simulink model "uz_interlockDeadtime2L"  (R2023a)
settings: Solver=FixedStepDiscrete  StartTime=0.0  StopTime=0.003  RelTol=1e-3
undefined symbols (not defined in the file or in its folder): f_FPGA_clk, T_FPGA_clk
libraries: simulink x3, hdlsllib x3
(part 2 of 2)

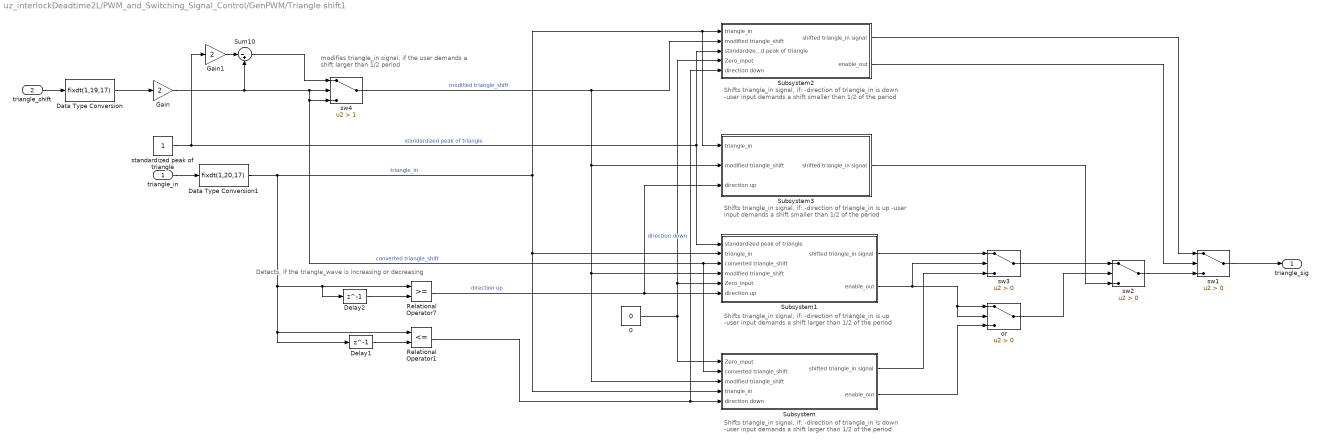
== system uz_interlockDeadtime2L/PWM_and_Switching_Signal_Control/GenPWM/Triangle shift1 ==
  note: modifies triangle_in signal,
      | if the user demands a shift larger than 1/2 period
  note: Detects, if the triangle_wave is increasing or decreasing
  note: Shifts triangle_in signal, if:
      | -direction of triangle_in is down
      | -user input demands a shift larger than 1/2 of the period
  note: Shifts triangle_in signal, if:
      | -direction of triangle_in is up
      | -user input demands a shift larger than 1/2 of the period
  note: Shifts triangle_in signal, if:
      | -direction of triangle_in is up
      | -user input demands a shift smaller than 1/2 of the period
  note: Shifts triangle_in signal, if:
      | -direction of triangle_in is down
      | -user input demands a shift smaller than 1/2 of the period
  triangle_in : Inport
  triangle_shift : Inport  Port=2
  0 : Constant  Value=0  OutDataTypeStr=boolean  SampleTime=T_FPGA_clk
  Data Type Conversion : DataTypeConversion  OutDataTypeStr=fixdt(1,19,17)  SaturateOnIntegerOverflow=off  RndMeth=Floor
  Data Type Conversion1 : DataTypeConversion  OutDataTypeStr=fixdt(1,20,17)  SaturateOnIntegerOverflow=off  RndMeth=Floor
  Delay1 : Delay  DelayLength=1
  Delay2 : Delay  DelayLength=1
  Gain : Gain  Gain=2  OutDataTypeStr=fixdt(1,20,17)
  Gain1 : Gain  Gain=2  OutDataTypeStr=fixdt(1,20,17)
  Relational Operator1 : RelationalOperator  Operator=<=  OutDataTypeStr=boolean  InputSameDT=off
  Relational Operator7 : RelationalOperator  OutDataTypeStr=boolean  InputSameDT=off
  Subsystem : Subsystem
  Subsystem1 : Subsystem
  Subsystem2 : Subsystem
  Subsystem3 : Subsystem
  Sum10 : Sum  Inputs=|-+  OutDataTypeStr=fixdt(1,20,17)
  or : Switch  Criteria=u2 > Threshold  SaturateOnIntegerOverflow=off  InputSameDT=off
  standardized peak of triangle : Constant  OutDataTypeStr=fixdt(0,21,17)  SampleTime=T_FPGA_clk
  sw1 : Switch  Criteria=u2 > Threshold  OutDataTypeStr=fixdt(1,18,16)  SaturateOnIntegerOverflow=off  InputSameDT=off
  sw2 : Switch  Criteria=u2 > Threshold  SaturateOnIntegerOverflow=off  InputSameDT=off
  sw3 : Switch  Criteria=u2 > Threshold  SaturateOnIntegerOverflow=off  InputSameDT=off
  sw4 : Switch  Criteria=u2 > Threshold  Threshold=1  OutDataTypeStr=fixdt(1,20,17)  SaturateOnIntegerOverflow=off  InputSameDT=off
  triangle_sig : Outport  VectorParamsAs1DForOutWhenUnconnected=off
  wires:
  Delay2/1 -> Relational Operator7/2
  Data Type Conversion1/1 -> Subsystem3/1(triangle_in), Subsystem2/1(triangle_in), Subsystem/4(triangle_in), Subsystem1/2(triangle_in), Relational Operator1/1, Delay1/1, Delay2/1, Relational Operator7/1  "triangle_in"
  sw3/1 -> sw2/1
  Relational Operator7/1 -> Subsystem1/6(direction up), Subsystem3/3(direction up)  "direction up"
  or/1 -> sw2/2
  sw4/1 -> Subsystem3/2(modified triangle_shift), Subsystem/3(modified triangle_shift), Subsystem1/4(modified triangle_shift), Subsystem2/2(modified triangle_shift)  "modified triangle_shift"
  Gain/1 -> Sum10/2, Subsystem/2(converted triangle_shift), Subsystem1/3(converted triangle_shift), sw4/3, sw4/2  "converted triangle_shift"
  Sum10/1 -> sw4/1
  sw1/1 -> triangle_sig/1
  standardized peak of triangle/1 -> Subsystem2/3(standardized peak of triangle), Subsystem1/1(standardized peak of triangle), Gain1/1  "standardized peak of triangle"
  triangle_shift/1 -> Data Type Conversion/1
  Gain1/1 -> Sum10/1
  sw2/1 -> sw1/3
  Data Type Conversion/1 -> Gain/1
  triangle_in/1 -> Data Type Conversion1/1
  Relational Operator1/1 -> Subsystem/5(direction down), Subsystem2/5(direction down)  "direction down"
  Delay1/1 -> Relational Operator1/2
  0/1 -> Subsystem2/4(Zero_input), Subsystem1/5(Zero_input), Subsystem/1(Zero_input)
  Subsystem/1(shifted triangle_in signal) -> sw3/3
  Subsystem/2(enable_out) -> or/3
  Subsystem1/2(enable_out) -> or/2, or/1, sw3/2
  Subsystem1/1(shifted triangle_in signal) -> sw3/1
  Subsystem2/1(shifted triangle_in signal) -> sw1/1
  Subsystem2/2(enable_out) -> sw1/2
  Subsystem3/1(shifted triangle_in signal) -> sw2/3

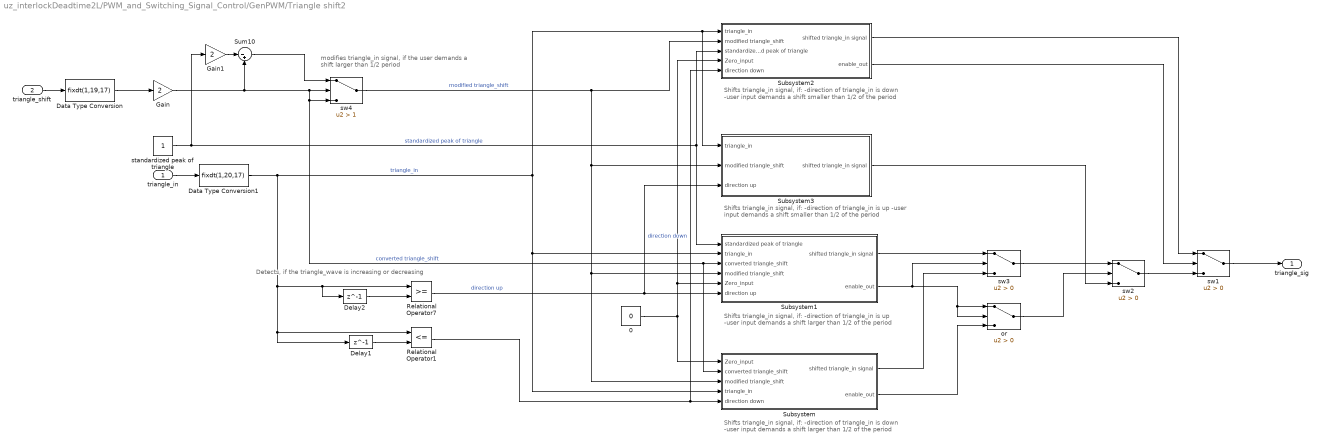
== system uz_interlockDeadtime2L/PWM_and_Switching_Signal_Control/GenPWM/Triangle shift2 ==
  note: modifies triangle_in signal,
      | if the user demands a shift larger than 1/2 period
  note: Detects, if the triangle_wave is increasing or decreasing
  note: Shifts triangle_in signal, if:
      | -direction of triangle_in is down
      | -user input demands a shift larger than 1/2 of the period
  note: Shifts triangle_in signal, if:
      | -direction of triangle_in is up
      | -user input demands a shift larger than 1/2 of the period
  note: Shifts triangle_in signal, if:
      | -direction of triangle_in is up
      | -user input demands a shift smaller than 1/2 of the period
  note: Shifts triangle_in signal, if:
      | -direction of triangle_in is down
      | -user input demands a shift smaller than 1/2 of the period
  triangle_in : Inport
  triangle_shift : Inport  Port=2
  0 : Constant  Value=0  OutDataTypeStr=boolean  SampleTime=T_FPGA_clk
  Data Type Conversion : DataTypeConversion  OutDataTypeStr=fixdt(1,19,17)  SaturateOnIntegerOverflow=off  RndMeth=Floor
  Data Type Conversion1 : DataTypeConversion  OutDataTypeStr=fixdt(1,20,17)  SaturateOnIntegerOverflow=off  RndMeth=Floor
  Delay1 : Delay  DelayLength=1
  Delay2 : Delay  DelayLength=1
  Gain : Gain  Gain=2  OutDataTypeStr=fixdt(1,20,17)
  Gain1 : Gain  Gain=2  OutDataTypeStr=fixdt(1,20,17)
  Relational Operator1 : RelationalOperator  Operator=<=  OutDataTypeStr=boolean  InputSameDT=off
  Relational Operator7 : RelationalOperator  OutDataTypeStr=boolean  InputSameDT=off
  Subsystem : Subsystem
  Subsystem1 : Subsystem
  Subsystem2 : Subsystem
  Subsystem3 : Subsystem
  Sum10 : Sum  Inputs=|-+  OutDataTypeStr=fixdt(1,20,17)
  or : Switch  Criteria=u2 > Threshold  SaturateOnIntegerOverflow=off  InputSameDT=off
  standardized peak of triangle : Constant  OutDataTypeStr=fixdt(0,21,17)  SampleTime=T_FPGA_clk
  sw1 : Switch  Criteria=u2 > Threshold  OutDataTypeStr=fixdt(1,18,16)  SaturateOnIntegerOverflow=off  InputSameDT=off
  sw2 : Switch  Criteria=u2 > Threshold  SaturateOnIntegerOverflow=off  InputSameDT=off
  sw3 : Switch  Criteria=u2 > Threshold  SaturateOnIntegerOverflow=off  InputSameDT=off
  sw4 : Switch  Criteria=u2 > Threshold  Threshold=1  OutDataTypeStr=fixdt(1,20,17)  SaturateOnIntegerOverflow=off  InputSameDT=off
  triangle_sig : Outport  VectorParamsAs1DForOutWhenUnconnected=off
  wires:
  Delay2/1 -> Relational Operator7/2
  Data Type Conversion1/1 -> Subsystem3/1(triangle_in), Subsystem2/1(triangle_in), Subsystem/4(triangle_in), Subsystem1/2(triangle_in), Relational Operator1/1, Delay1/1, Delay2/1, Relational Operator7/1  "triangle_in"
  sw3/1 -> sw2/1
  Relational Operator7/1 -> Subsystem1/6(direction up), Subsystem3/3(direction up)  "direction up"
  or/1 -> sw2/2
  sw4/1 -> Subsystem3/2(modified triangle_shift), Subsystem/3(modified triangle_shift), Subsystem1/4(modified triangle_shift), Subsystem2/2(modified triangle_shift)  "modified triangle_shift"
  Gain/1 -> Sum10/2, Subsystem/2(converted triangle_shift), Subsystem1/3(converted triangle_shift), sw4/3, sw4/2  "converted triangle_shift"
  Sum10/1 -> sw4/1
  sw1/1 -> triangle_sig/1
  standardized peak of triangle/1 -> Subsystem2/3(standardized peak of triangle), Subsystem1/1(standardized peak of triangle), Gain1/1  "standardized peak of triangle"
  triangle_shift/1 -> Data Type Conversion/1
  Gain1/1 -> Sum10/1
  sw2/1 -> sw1/3
  Data Type Conversion/1 -> Gain/1
  triangle_in/1 -> Data Type Conversion1/1
  Relational Operator1/1 -> Subsystem/5(direction down), Subsystem2/5(direction down)  "direction down"
  Delay1/1 -> Relational Operator1/2
  0/1 -> Subsystem2/4(Zero_input), Subsystem1/5(Zero_input), Subsystem/1(Zero_input)
  Subsystem/1(shifted triangle_in signal) -> sw3/3
  Subsystem/2(enable_out) -> or/3
  Subsystem1/2(enable_out) -> or/2, or/1, sw3/2
  Subsystem1/1(shifted triangle_in signal) -> sw3/1
  Subsystem2/1(shifted triangle_in signal) -> sw1/1
  Subsystem2/2(enable_out) -> sw1/2
  Subsystem3/1(shifted triangle_in signal) -> sw2/3

== system uz_interlockDeadtime2L/PWM_and_Switching_Signal_Control/GenPWM/Triangle shift/Subsystem ==
  note: AND block replaced with
      | switches for better performance
  Zero_input : Inport
  converted triangle_shift : Inport  Port=2
  modified triangle_shift : Inport  Port=3
  triangle_in : Inport  Port=4
  direction down : Inport  Port=5
  Relational Operator11 : RelationalOperator  Operator=<=  OutDataTypeStr=boolean  InputSameDT=off
  Sum8 : Sum  Inputs=|-+
  Unary Minus : UnaryMinus
  and2_1 : Switch  Criteria=u2 > Threshold  SaturateOnIntegerOverflow=off  InputSameDT=off
  and2_2 : Switch  Criteria=u2 > Threshold  SaturateOnIntegerOverflow=off  InputSameDT=off
  shifted triangle_in signal : Outport
  enable_out : Outport  Port=2
  wires:
  direction down/1 -> and2_2/2
  Zero_input/1 -> and2_1/3, and2_2/3
  Relational Operator11/1 -> and2_1/2
  and2_1/1 -> and2_2/1
  Sum8/1 -> shifted triangle_in signal/1
  Unary Minus/1 -> Sum8/2, Relational Operator11/2
  triangle_in/1 -> Sum8/1, Relational Operator11/1
  converted triangle_shift/1 -> and2_1/1
  and2_2/1 -> enable_out/1
  modified triangle_shift/1 -> Unary Minus/1

== system uz_interlockDeadtime2L/PWM_and_Switching_Signal_Control/GenPWM/Triangle shift/Subsystem1 ==
  note: AND block replaced with
      | switches for better performance
  note: AND block replaced with
      | switches for better performance
  standardized peak of triangle : Inport
  triangle_in : Inport  Port=2
  converted triangle_shift : Inport  Port=3
  modified triangle_shift : Inport  Port=4
  Zero_input : Inport  Port=5
  direction up : Inport  Port=6
  Relational Operator2 : RelationalOperator  OutDataTypeStr=boolean  InputSameDT=off
  Sum11 : Sum  Inputs=++-  OutDataTypeStr=fixdt(1,21,17)
  Sum6 : Sum  Inputs=++|
  and1_1 : Switch  Criteria=u2 > Threshold  SaturateOnIntegerOverflow=off  InputSameDT=off
  and1_2 : Switch  Criteria=u2 > Threshold  SaturateOnIntegerOverflow=off  InputSameDT=off
  shifted triangle_in signal : Outport
  enable_out : Outport  Port=2
  wires:
  Sum11/1 -> shifted triangle_in signal/1
  Sum6/1 -> Relational Operator2/2, Sum11/2
  and1_1/1 -> and1_2/1
  Relational Operator2/1 -> and1_1/2
  Zero_input/1 -> and1_2/3, and1_1/3
  standardized peak of triangle/1 -> Sum6/2, Sum11/1
  and1_2/1 -> enable_out/1
  converted triangle_shift/1 -> and1_1/1
  direction up/1 -> and1_2/2
  triangle_in/1 -> Relational Operator2/1, Sum11/3
  modified triangle_shift/1 -> Sum6/1

== system uz_interlockDeadtime2L/PWM_and_Switching_Signal_Control/GenPWM/Triangle shift/Subsystem2 ==
  triangle_in : Inport
  modified triangle_shift : Inport  Port=2
  standardized peak of triangle : Inport  Port=3
  Zero_input : Inport  Port=4
  direction down : Inport  Port=5
  Relational Operator9 : RelationalOperator  OutDataTypeStr=boolean  InputSameDT=off
  Sum1 : Sum  Inputs=|-+
  Sum5 : Sum  Inputs=++-  OutDataTypeStr=fixdt(1,21,17)
  and : Switch  Criteria=u2 > Threshold  SaturateOnIntegerOverflow=off  InputSameDT=off
  shifted triangle_in signal : Outport
  enable_out : Outport  Port=2
  wires:
  standardized peak of triangle/1 -> Sum1/2, Sum5/2
  Zero_input/1 -> and/3
  Sum1/1 -> Relational Operator9/2, Sum5/1
  Relational Operator9/1 -> and/1
  direction down/1 -> and/2
  and/1 -> enable_out/1
  triangle_in/1 -> Relational Operator9/1, Sum5/3
  Sum5/1 -> shifted triangle_in signal/1
  modified triangle_shift/1 -> Sum1/1

== system uz_interlockDeadtime2L/PWM_and_Switching_Signal_Control/GenPWM/Triangle shift/Subsystem3 ==
  triangle_in : Inport
  modified triangle_shift : Inport  Port=2
  direction up : Inport  Port=3
  Relational Operator6 : RelationalOperator  Operator=<=  OutDataTypeStr=boolean  InputSameDT=off
  Sum2 : Sum  Inputs=|-+
  Sum3 : Sum  Inputs=|+-
  Sum4 : Sum  Inputs=|++
  Switch3 : Switch  Criteria=u2 > Threshold  SaturateOnIntegerOverflow=off  InputSameDT=off
  sw : Switch  Criteria=u2 > Threshold  SaturateOnIntegerOverflow=off  InputSameDT=off
  shifted triangle_in signal : Outport
  wires:
  Sum4/1 -> sw/3
  modified triangle_shift/1 -> Sum4/1, Sum3/2, Sum2/2, Relational Operator6/2
  Switch3/1 -> sw/1
  Sum3/1 -> Switch3/3
  Sum2/1 -> Switch3/1
  sw/1 -> shifted triangle_in signal/1
  Relational Operator6/1 -> Switch3/2
  direction up/1 -> sw/2
  triangle_in/1 -> Relational Operator6/1, Sum3/1, Sum2/1, Sum4/2

== system uz_interlockDeadtime2L/PWM_and_Switching_Signal_Control/GenPWM/Triangle shift1/Subsystem ==
  note: AND block replaced with
      | switches for better performance
  Zero_input : Inport
  converted triangle_shift : Inport  Port=2
  modified triangle_shift : Inport  Port=3
  triangle_in : Inport  Port=4
  direction down : Inport  Port=5
  Relational Operator11 : RelationalOperator  Operator=<=  OutDataTypeStr=boolean  InputSameDT=off
  Sum8 : Sum  Inputs=|-+
  Unary Minus : UnaryMinus
  and2_1 : Switch  Criteria=u2 > Threshold  SaturateOnIntegerOverflow=off  InputSameDT=off
  and2_2 : Switch  Criteria=u2 > Threshold  SaturateOnIntegerOverflow=off  InputSameDT=off
  shifted triangle_in signal : Outport
  enable_out : Outport  Port=2
  wires:
  direction down/1 -> and2_2/2
  Zero_input/1 -> and2_1/3, and2_2/3
  Relational Operator11/1 -> and2_1/2
  and2_1/1 -> and2_2/1
  Sum8/1 -> shifted triangle_in signal/1
  Unary Minus/1 -> Sum8/2, Relational Operator11/2
  triangle_in/1 -> Sum8/1, Relational Operator11/1
  converted triangle_shift/1 -> and2_1/1
  and2_2/1 -> enable_out/1
  modified triangle_shift/1 -> Unary Minus/1

== system uz_interlockDeadtime2L/PWM_and_Switching_Signal_Control/GenPWM/Triangle shift1/Subsystem1 ==
  note: AND block replaced with
      | switches for better performance
  note: AND block replaced with
      | switches for better performance
  standardized peak of triangle : Inport
  triangle_in : Inport  Port=2
  converted triangle_shift : Inport  Port=3
  modified triangle_shift : Inport  Port=4
  Zero_input : Inport  Port=5
  direction up : Inport  Port=6
  Relational Operator2 : RelationalOperator  OutDataTypeStr=boolean  InputSameDT=off
  Sum11 : Sum  Inputs=++-  OutDataTypeStr=fixdt(1,21,17)
  Sum6 : Sum  Inputs=++|
  and1_1 : Switch  Criteria=u2 > Threshold  SaturateOnIntegerOverflow=off  InputSameDT=off
  and1_2 : Switch  Criteria=u2 > Threshold  SaturateOnIntegerOverflow=off  InputSameDT=off
  shifted triangle_in signal : Outport
  enable_out : Outport  Port=2
  wires:
  Sum11/1 -> shifted triangle_in signal/1
  Sum6/1 -> Relational Operator2/2, Sum11/2
  and1_1/1 -> and1_2/1
  Relational Operator2/1 -> and1_1/2
  Zero_input/1 -> and1_2/3, and1_1/3
  standardized peak of triangle/1 -> Sum6/2, Sum11/1
  and1_2/1 -> enable_out/1
  converted triangle_shift/1 -> and1_1/1
  direction up/1 -> and1_2/2
  triangle_in/1 -> Relational Operator2/1, Sum11/3
  modified triangle_shift/1 -> Sum6/1

== system uz_interlockDeadtime2L/PWM_and_Switching_Signal_Control/GenPWM/Triangle shift1/Subsystem2 ==
  triangle_in : Inport
  modified triangle_shift : Inport  Port=2
  standardized peak of triangle : Inport  Port=3
  Zero_input : Inport  Port=4
  direction down : Inport  Port=5
  Relational Operator9 : RelationalOperator  OutDataTypeStr=boolean  InputSameDT=off
  Sum1 : Sum  Inputs=|-+
  Sum5 : Sum  Inputs=++-  OutDataTypeStr=fixdt(1,21,17)
  and : Switch  Criteria=u2 > Threshold  SaturateOnIntegerOverflow=off  InputSameDT=off
  shifted triangle_in signal : Outport
  enable_out : Outport  Port=2
  wires:
  standardized peak of triangle/1 -> Sum1/2, Sum5/2
  Zero_input/1 -> and/3
  Sum1/1 -> Relational Operator9/2, Sum5/1
  Relational Operator9/1 -> and/1
  direction down/1 -> and/2
  and/1 -> enable_out/1
  triangle_in/1 -> Relational Operator9/1, Sum5/3
  Sum5/1 -> shifted triangle_in signal/1
  modified triangle_shift/1 -> Sum1/1

== system uz_interlockDeadtime2L/PWM_and_Switching_Signal_Control/GenPWM/Triangle shift1/Subsystem3 ==
  triangle_in : Inport
  modified triangle_shift : Inport  Port=2
  direction up : Inport  Port=3
  Relational Operator6 : RelationalOperator  Operator=<=  OutDataTypeStr=boolean  InputSameDT=off
  Sum2 : Sum  Inputs=|-+
  Sum3 : Sum  Inputs=|+-
  Sum4 : Sum  Inputs=|++
  Switch3 : Switch  Criteria=u2 > Threshold  SaturateOnIntegerOverflow=off  InputSameDT=off
  sw : Switch  Criteria=u2 > Threshold  SaturateOnIntegerOverflow=off  InputSameDT=off
  shifted triangle_in signal : Outport
  wires:
  Sum4/1 -> sw/3
  modified triangle_shift/1 -> Sum4/1, Sum3/2, Sum2/2, Relational Operator6/2
  Switch3/1 -> sw/1
  Sum3/1 -> Switch3/3
  Sum2/1 -> Switch3/1
  sw/1 -> shifted triangle_in signal/1
  Relational Operator6/1 -> Switch3/2
  direction up/1 -> sw/2
  triangle_in/1 -> Relational Operator6/1, Sum3/1, Sum2/1, Sum4/2

== system uz_interlockDeadtime2L/PWM_and_Switching_Signal_Control/GenPWM/Triangle shift2/Subsystem ==
  note: AND block replaced with
      | switches for better performance
  Zero_input : Inport
  converted triangle_shift : Inport  Port=2
  modified triangle_shift : Inport  Port=3
  triangle_in : Inport  Port=4
  direction down : Inport  Port=5
  Relational Operator11 : RelationalOperator  Operator=<=  OutDataTypeStr=boolean  InputSameDT=off
  Sum8 : Sum  Inputs=|-+
  Unary Minus : UnaryMinus
  and2_1 : Switch  Criteria=u2 > Threshold  SaturateOnIntegerOverflow=off  InputSameDT=off
  and2_2 : Switch  Criteria=u2 > Threshold  SaturateOnIntegerOverflow=off  InputSameDT=off
  shifted triangle_in signal : Outport
  enable_out : Outport  Port=2
  wires:
  direction down/1 -> and2_2/2
  Zero_input/1 -> and2_1/3, and2_2/3
  Relational Operator11/1 -> and2_1/2
  and2_1/1 -> and2_2/1
  Sum8/1 -> shifted triangle_in signal/1
  Unary Minus/1 -> Sum8/2, Relational Operator11/2
  triangle_in/1 -> Sum8/1, Relational Operator11/1
  converted triangle_shift/1 -> and2_1/1
  and2_2/1 -> enable_out/1
  modified triangle_shift/1 -> Unary Minus/1

== system uz_interlockDeadtime2L/PWM_and_Switching_Signal_Control/GenPWM/Triangle shift2/Subsystem1 ==
  note: AND block replaced with
      | switches for better performance
  note: AND block replaced with
      | switches for better performance
  standardized peak of triangle : Inport
  triangle_in : Inport  Port=2
  converted triangle_shift : Inport  Port=3
  modified triangle_shift : Inport  Port=4
  Zero_input : Inport  Port=5
  direction up : Inport  Port=6
  Relational Operator2 : RelationalOperator  OutDataTypeStr=boolean  InputSameDT=off
  Sum11 : Sum  Inputs=++-  OutDataTypeStr=fixdt(1,21,17)
  Sum6 : Sum  Inputs=++|
  and1_1 : Switch  Criteria=u2 > Threshold  SaturateOnIntegerOverflow=off  InputSameDT=off
  and1_2 : Switch  Criteria=u2 > Threshold  SaturateOnIntegerOverflow=off  InputSameDT=off
  shifted triangle_in signal : Outport
  enable_out : Outport  Port=2
  wires:
  Sum11/1 -> shifted triangle_in signal/1
  Sum6/1 -> Relational Operator2/2, Sum11/2
  and1_1/1 -> and1_2/1
  Relational Operator2/1 -> and1_1/2
  Zero_input/1 -> and1_2/3, and1_1/3
  standardized peak of triangle/1 -> Sum6/2, Sum11/1
  and1_2/1 -> enable_out/1
  converted triangle_shift/1 -> and1_1/1
  direction up/1 -> and1_2/2
  triangle_in/1 -> Relational Operator2/1, Sum11/3
  modified triangle_shift/1 -> Sum6/1

== system uz_interlockDeadtime2L/PWM_and_Switching_Signal_Control/GenPWM/Triangle shift2/Subsystem2 ==
  triangle_in : Inport
  modified triangle_shift : Inport  Port=2
  standardized peak of triangle : Inport  Port=3
  Zero_input : Inport  Port=4
  direction down : Inport  Port=5
  Relational Operator9 : RelationalOperator  OutDataTypeStr=boolean  InputSameDT=off
  Sum1 : Sum  Inputs=|-+
  Sum5 : Sum  Inputs=++-  OutDataTypeStr=fixdt(1,21,17)
  and : Switch  Criteria=u2 > Threshold  SaturateOnIntegerOverflow=off  InputSameDT=off
  shifted triangle_in signal : Outport
  enable_out : Outport  Port=2
  wires:
  standardized peak of triangle/1 -> Sum1/2, Sum5/2
  Zero_input/1 -> and/3
  Sum1/1 -> Relational Operator9/2, Sum5/1
  Relational Operator9/1 -> and/1
  direction down/1 -> and/2
  and/1 -> enable_out/1
  triangle_in/1 -> Relational Operator9/1, Sum5/3
  Sum5/1 -> shifted triangle_in signal/1
  modified triangle_shift/1 -> Sum1/1

== system uz_interlockDeadtime2L/PWM_and_Switching_Signal_Control/GenPWM/Triangle shift2/Subsystem3 ==
  triangle_in : Inport
  modified triangle_shift : Inport  Port=2
  direction up : Inport  Port=3
  Relational Operator6 : RelationalOperator  Operator=<=  OutDataTypeStr=boolean  InputSameDT=off
  Sum2 : Sum  Inputs=|-+
  Sum3 : Sum  Inputs=|+-
  Sum4 : Sum  Inputs=|++
  Switch3 : Switch  Criteria=u2 > Threshold  SaturateOnIntegerOverflow=off  InputSameDT=off
  sw : Switch  Criteria=u2 > Threshold  SaturateOnIntegerOverflow=off  InputSameDT=off
  shifted triangle_in signal : Outport
  wires:
  Sum4/1 -> sw/3
  modified triangle_shift/1 -> Sum4/1, Sum3/2, Sum2/2, Relational Operator6/2
  Switch3/1 -> sw/1
  Sum3/1 -> Switch3/3
  Sum2/1 -> Switch3/1
  sw/1 -> shifted triangle_in signal/1
  Relational Operator6/1 -> Switch3/2
  direction up/1 -> sw/2
  triangle_in/1 -> Relational Operator6/1, Sum3/1, Sum2/1, Sum4/2
